simulink model "ksp_zad17"  (Simulink 7.1)
settings: Solver=ode45  SolverMode=SingleTasking  StartTime=0.0  StopTime=20.0  MaxStep=0.01  RelTol=0.001  AbsTol=1e-6
settings Model: Creator=Slavi  LastModifiedBy=Slavi
settings SolverCC: InitialStep=0.01
settings DataIOCC: LimitDataPoints=off
settings OptimizationCC: BlockReduction=off  BooleanDataType=off
settings DebuggingCC: SaveWithParameterizedLinksMsg=none  SignalResolutionControl=TryResolveAllWithWarning  SolverPrmCheckMsg=none  MultiTaskDSMMsg=warning  MultiTaskCondExecSysMsg=none  StrictBusMsg=None
settings HardwareCC: TargetUnknown=on
settings RTWCC: IncludeERTFirstTime=on

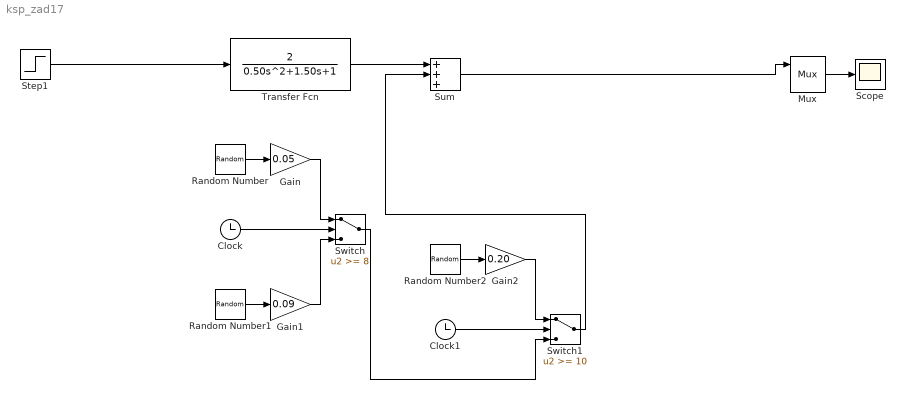
== system ksp_zad17 ==
  Clock : Clock
      settings: Decimation=10
  Clock1 : Clock
      settings: Decimation=10
  Gain : Gain  Gain=0.05  SaturateOnIntegerOverflow=on  OutDataTypeStr=Inherit: Same as input  ParamDataTypeStr=Inherit: Same as input
  Gain1 : Gain  Gain=0.09  SaturateOnIntegerOverflow=on  OutDataTypeStr=Inherit: Same as input  ParamDataTypeStr=Inherit: Same as input
  Gain2 : Gain  Gain=0.20  SaturateOnIntegerOverflow=on  OutDataTypeStr=Inherit: Same as input  ParamDataTypeStr=Inherit: Same as input
  Mux : Mux  Inputs=3
  Random Number : RandomNumber  SampleTime=0
  Random Number1 : RandomNumber  SampleTime=0
  Random Number2 : RandomNumber  SampleTime=0
  Scope : Scope
      settings: TickLabels=on  YMin=-4  YMax=4  DataFormat=Array
  Step1 : Step  Time=0
  Sum : Sum  Inputs=+++  SaturateOnIntegerOverflow=on  InputSameDT=on  OutDataTypeStr=Inherit: Same as first input
  Switch : Switch  Threshold=8  SaturateOnIntegerOverflow=on  InputSameDT=on
  Switch1 : Switch  Threshold=10  SaturateOnIntegerOverflow=on  InputSameDT=on
  Transfer Fcn : TransferFcn  Numerator=[2]  Denominator=[0.50 1.50 1]
  wires:
  Step1/1 -> Transfer Fcn/1
  Mux/1 -> Scope/1
  Clock/1 -> Switch/2
  Transfer Fcn/1 -> Sum/1
  Sum/1 -> Mux/1
  Random Number/1 -> Gain/1
  Gain/1 -> Switch/1
  Random Number1/1 -> Gain1/1
  Gain1/1 -> Switch/3
  Clock1/1 -> Switch1/2
  Gain2/1 -> Switch1/1
  Random Number2/1 -> Gain2/1
  Switch/1 -> Switch1/3
  Switch1/1 -> Sum/2
